simulink model "PV_array_final"  (R2019a)
settings: Solver=VariableStepAuto  StartTime=0.0  StopTime=1  FixedStep=5e-6  RelTol=1e-3
libraries: powerlib x9, powerlib_meascontrol x3, re_lib x1
settings Model: Creator=SUMANTH  LastModifiedBy=SUMANTH
settings SolverCC: AlgebraicLoopSolver=LineSearch
settings DataIOCC: ReturnWorkspaceOutputs=off  LoggingToFile=on

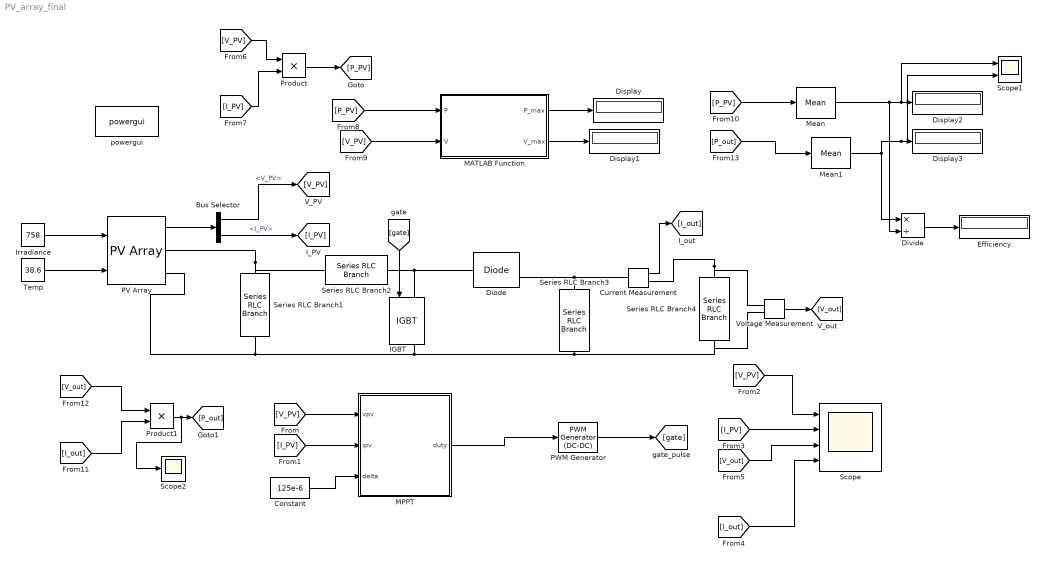
== system PV_array_final ==
  Bus Selector : BusSelector  OutputSignals=V_PV,I_PV
  Constant : Constant  Value=125e-6
  Current Measurement : powerlib/Measurements/Current Measurement  PhasorSimulation=off  OutputType=Complex  PSBequivalent=0
      settings: SourceProductName=Simscape Electrical
  Diode : powerlib/Power Electronics/Diode  Ron=0.001  Lon=0  Vf=0.8  IC=0  UseSnubber=0  Rs=500  Cs=250e-9  Measurements=on
      settings: SourceProductName=Simscape Electrical
  Display{,1..3} (4 alike) : Display
  Divide : Product  Inputs=*/
  Efficiency : Display
  IGBT : powerlib/Power Electronics/IGBT  Ron=0.001  Lon=0  Vf=1  Tf=1e-6  Tt=2e-6  IC=0  Rs=1e5  Cs=inf  Measurements=on
      settings: SourceProductName=Simscape Electrical
  Irradiance : Constant  Value=758
  MATLAB Function : MATLAB Function  TreatAsAtomicUnit=on
  MPPT : MATLAB Function  TreatAsAtomicUnit=on
  Mean : powerlib_meascontrol/Measurements/Mean  Freq=60  Vinit=0  Ts=0
      settings: SourceProductName=Simscape Electrical
  Mean1 : powerlib_meascontrol/Measurements/Mean  Freq=60  Vinit=0  Ts=0
      settings: SourceProductName=Simscape Electrical
  PV Array : re_lib/Solar/PV Array  Npar=2  Nser=2  PlotType=array @ 25 deg.C & specified irradiances  S_vec="[ 1000  500  100 ]"  Temp_C_vec="[ 45 25  ]"  ModuleName=1Soltech 1STH-215-P  PlotWhenSelected=off  Pm=213.15  Ncell=60  Voc=36.3  Isc=7.84  Vm=29  Im=7.35  beta_Voc_pc=-0.36099  alpha_Isc_pc=0.102  beta_Voc=-0.13104  alpha_Isc=0.007997  IL=7.8649  I0=2.9259e-10  nI=0.98117  Rsh=313.3991  Rs=0.39383  BAL=off  Tc=1e-6  Tfilter=1e-6
      settings: SourceProductName=Simscape Electrical
  PWM Generator : powerlib_meascontrol/Pulse & Signal Generators/PWM Generator (DC-DC)  Fsw=5000  Ts=0
      settings: SourceProductName=Simscape Electrical
  Product : Product
  Product1 : Product
  Scope : Scope  NumInputPorts=4
  Scope1 : Scope  NumInputPorts=2
  Scope2 : Scope
  Series RLC Branch1 : powerlib/Elements/Series RLC Branch  LConnTagsString=__new0  RConnTagsString=__new0  BranchType=C  Resistance=1  Inductance=1e-3  SetiL0=off  InitialCurrent=0  Capacitance=1e-4  Setx0=off  InitialVoltage=0  Measurements=None
      settings: SourceProductName=Simscape Electrical
  Series RLC Branch2 : powerlib/Elements/Series RLC Branch  LConnTagsString=__new0  RConnTagsString=__new0  BranchType=L  Resistance=1  Inductance=4.44e-3  SetiL0=off  InitialCurrent=0  Capacitance=1e-6  Setx0=off  InitialVoltage=0  Measurements=None
      settings: SourceProductName=Simscape Electrical
  Series RLC Branch3 : powerlib/Elements/Series RLC Branch  LConnTagsString=__new0  RConnTagsString=__new0  BranchType=C  Resistance=1  Inductance=1e-3  SetiL0=off  InitialCurrent=0  Capacitance=9.09e-5  Setx0=off  InitialVoltage=0  Measurements=None
      settings: SourceProductName=Simscape Electrical
  Series RLC Branch4 : powerlib/Elements/Series RLC Branch  LConnTagsString=__new0  RConnTagsString=__new0  BranchType=R  Resistance=16.22  Inductance=1e-3  SetiL0=off  InitialCurrent=0  Capacitance=1e-6  Setx0=off  InitialVoltage=0  Measurements=None
      settings: SourceProductName=Simscape Electrical
  Temp : Constant  Value=38.6
  Voltage Measurement : powerlib/Measurements/Voltage Measurement  PhasorSimulation=off  OutputType=Complex  PSBequivalent=0
      settings: SourceProductName=Simscape Electrical
  powergui : powerlib/powergui  Priority=1  SimulationMode=Continuous  SampleTime=5e-6  frequency=60  Iterations=50  frequencyindice=0  Pbase=100e6  ErrMax=1e-4  UnitsV=kV  UnitsW=MW  buscounter=0  FunctionMessages=off  echomessages=off  EnableUseOfTLC=off  CurrentSourceSwitches=off  DisableSnubberDevices=off  DisableRonSwitches=off  DisableVfSwitches=off  DisplayEquations=off  AutomaticDiscreteSolvers=off  SolverType=Tustin/Backward Euler (TBE)  Interpol=off  ExternalGateDelay=off  methode=off  Ts=100  x0status=blocks  SPID=on  SwTol=0  HookPort=off  NonlinearTolerance=0  nMaxIteration=15  ContinueOnMaxIteration=off  RestoreLinks=warning  ResistiveCurrentMeasurement=off  Frange=[0:2:500]  Ylog=off  Xlog=on  ShowGrid=off  save=off  variable=ZData  structure=ScopeData2  ZoomFFT=on  StartTime=0.0  cycles=1  DisplayStyle=2  fundamental=60  FreqAxis=off  MaxFrequency=1000  frequencyindicesteady=1  RmsSteady=1  display=off
      settings: SourceProductName=Simscape Electrical
  wires:
  Irradiance/1 -> PV Array/1
  Temp/1 -> PV Array/2
  PV Array/1 -> Bus Selector/1
  Bus Selector/1 -> [V_PV]  "<V_PV>"
  Bus Selector/2 -> [I_PV]  "<I_PV>"
  Current Measurement/1 -> [I_out]
  Voltage Measurement/1 -> [V_out]
  [gate] -> IGBT/1
  PWM Generator/1 -> [gate]
  MPPT/1(duty) -> PWM Generator/1
  [V_PV] -> Scope/1
  [I_PV] -> Scope/2
  [I_out] -> Scope/4
  [V_out] -> Scope/3
  Constant/1 -> MPPT/3(delta)
  [I_PV] -> MPPT/2(ipv)
  [V_PV] -> MPPT/1(vpv)
  MATLAB Function/1(P_max) -> Display/1
  MATLAB Function/2(V_max) -> Display1/1
  [V_PV] -> Product/1
  [I_PV] -> Product/2
  Product/1 -> [P_PV]
  [P_PV] -> MATLAB Function/1(P)
  [V_PV] -> MATLAB Function/2(V)
  [V_out] -> Product1/1
  [I_out] -> Product1/2
  Product1/1 -> Scope2/1, [P_out]
  [P_PV] -> Mean/1
  [P_out] -> Mean1/1
  Mean1/1 -> Divide/1, Scope1/2, Display3/1
  Mean/1 -> Divide/2, Scope1/1, Display2/1
  Divide/1 -> Efficiency/1
  connections:
  PV Array/RConn1 -- Series RLC Branch2/LConn1 -- Series RLC Branch1/LConn1
  PV Array/RConn2 -- Voltage Measurement/LConn2 -- Series RLC Branch4/RConn1 -- Series RLC Branch3/RConn1 -- IGBT/RConn1 -- Series RLC Branch1/RConn1
  Series RLC Branch2/RConn1 -- Diode/LConn1 -- IGBT/LConn1
  Series RLC Branch3/LConn1 -- Current Measurement/LConn1 -- Diode/RConn1
  Series RLC Branch4/LConn1 -- Current Measurement/RConn1 -- Voltage Measurement/LConn1

== matlab function PV_array_final/MPPT ==
  settings: updateMethod=DISCRETE
  data: vpv input; duty output; ipv input; delta input
function duty = MPPT_algorithm(vpv,ipv,delta)


duty_init = 0.1;
% min and max value are used to limit duty between
% 0 and 0.85
duty_min=0;
duty_max=0.85;

persistent Vold Pold duty_old;
% persistent variable type can be store the data
% we need the old data by obtain difference
% between old and new value
if isempty(Vold)
    Vold=0;
    Pold=0;
    duty_old=duty_init;
end
P= vpv*ipv; % power
dV= vpv - Vold; % difference between old and new voltage
dP= P - Pold;% difference between old and new power

% the algorithm in below search the dP/dV=0
% if the derivative equal to zero
% duty will not change
% if old and new power not equal
% &
% pv voltage bigger than 30V
% the algorithm will works
if dP ~= 0 && vpv>30
    if dP < 0
        if dV < 0
            duty = duty_old - delta;
        else
            duty = duty_old + delta;
        end
    else
        if dV < 0
            duty = duty_old + delta;
        else
            duty = duty_old - delta;
        end
    end
else
    duty = duty_old;
end

%the below if limits the duty between min and max
if duty >= duty_max
    duty=duty_max;
elseif duty<duty_min
    duty=duty_min;
end

% stored data
duty_old=duty;
Vold=vpv;
Pold=P;

== matlab function PV_array_final/MATLAB Function ==
  settings: updateMethod=DISCRETE
  data: P input; P_max output; V input; V_max output
function [P_max, V_max] = max_value(P,V)

persistent Pprevious Vprevious

if isempty(Pprevious)
    Pprevious = 0;
    Vprevious = 0;
end

if (Pprevious > P)
    P_max = Pprevious;
    V_max = Vprevious;
else
    P_max = P;
    V_max = V;
end

Pprevious = P_max;
Vprevious = V_max;
